simulink model "UGV_cont"  (R2016b)
settings: Solver=VariableStepAuto  StartTime=0.0  StopTime=20  RelTol=1e-3
undefined symbols (not defined in the file): UGV_init
settings Model: Creator=nagym  LastModifiedBy=nagym
settings DataIOCC: ReturnWorkspaceOutputs=on
settings SFSimCC: SimUseLocalCustomCode=on
settings RTWCC: RTWUseLocalCustomCode=on

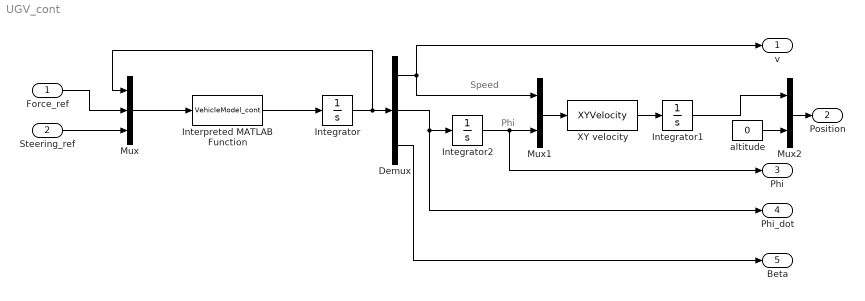
== system UGV_cont ==
  note: Phi
  note: Speed
  Force_ref : Inport
  Steering_ref : Inport  Port=2
  Demux : Demux  Outputs=3
  Integrator : Integrator  InitialCondition=UGV_init
  Integrator1 : Integrator  InitialCondition=[0 0]
  Integrator2 : Integrator
  Interpreted MATLAB Function : MATLABFcn  MATLABFcn=VehicleModel_cont  OutputDimensions=3
  Mux : Mux  Inputs=3
  Mux1 : Mux  Inputs=2
  Mux2 : Mux  Inputs=2
  XY velocity : MATLABFcn  MATLABFcn=XYVelocity  OutputDimensions=2
  altitude : Constant  Value=0
  v : Outport
  Position : Outport  Port=2
  Phi : Outport  Port=3
  Phi_dot : Outport  Port=4
  Beta : Outport  Port=5
  wires:
  Integrator/1 -> Demux/1, Mux/1
  Interpreted MATLAB Function/1 -> Integrator/1
  Mux/1 -> Interpreted MATLAB Function/1
  Demux/1 -> Mux1/1, v/1
  Integrator2/1 -> Phi/1, Mux1/2
  Demux/2 -> Phi_dot/1, Integrator2/1
  XY velocity/1 -> Integrator1/1
  Force_ref/1 -> Mux/2
  Steering_ref/1 -> Mux/3
  Mux1/1 -> XY velocity/1
  Demux/3 -> Beta/1
  Mux2/1 -> Position/1
  altitude/1 -> Mux2/2
  Integrator1/1 -> Mux2/1
